simulink model "IEEE9Buses"  (R2024b)
settings: Solver=FixedStepAuto  StartTime=0  StopTime=5  FixedStep=1e-6  RelTol=1e-3
values from neighbouring files (symbols this model uses):
  SG_D_1_D = 0.01056    [SG9_parameters.m]
  SG_D_1_EnableSaturation = 0    [SG9_parameters.m]
  SG_D_1_f0 = 60    [SG9_parameters.m]
  SG_D_1_H = 7.5    [SG9_parameters.m]
  SG_D_1_K_A = 20    [SG9_parameters.m]
  SG_D_1_K_E = 1.000000e+1    (= 10)    [SG9_parameters.m]
  SG_D_1_K_F = 2.363    [SG9_parameters.m]
  SG_D_1_K_s = 5    [SG9_parameters.m]
  SG_D_1_R_a = 0.001088    [SG9_parameters.m]
  SG_D_1_S_A = 1    [SG9_parameters.m]
  SG_D_1_S_B = 0.103    [SG9_parameters.m]
  SG_D_1_S_N = 10.659857    [SG9_parameters.m]
  SG_D_1_SpeedPara = 200    [SG9_parameters.m]
  SG_D_1_T_0 = 0.720173    [SG9_parameters.m]
  SG_D_1_T_1 = 0.3    [SG9_parameters.m]
  SG_D_1_T_2 = 0.05    [SG9_parameters.m]
  SG_D_1_T_3 = 0.02    [SG9_parameters.m]
  SG_D_1_T_4 = 0.005    [SG9_parameters.m]
  SG_D_1_T_A = 0.02    [SG9_parameters.m]
  SG_D_1_T_dd = 8.000000e+0    (= 8)    [SG9_parameters.m]
  SG_D_1_T_ddd = 0.04    [SG9_parameters.m]
  SG_D_1_T_E = 0.314    [SG9_parameters.m]
  SG_D_1_T_F = 0.35    [SG9_parameters.m]
  SG_D_1_T_qd = 0.8    [SG9_parameters.m]
  SG_D_1_T_qdd = 0.02    [SG9_parameters.m]
  SG_D_1_T_speed = 0.1    [SG9_parameters.m]
  SG_D_1_T_w = 0.5    [SG9_parameters.m]
  SG_D_1_V_ref = 1.990276    [SG9_parameters.m]
  SG_D_1_w_ref = 376.991118    [SG9_parameters.m]
  SG_D_1_x_d = 1.9    [SG9_parameters.m]
  SG_D_1_x_dd = 0.302    [SG9_parameters.m]
  SG_D_1_x_ddd = 0.204    [SG9_parameters.m]
  SG_D_1_x_l = 0.05    [SG9_parameters.m]
  SG_D_1_x_q = 1.3    [SG9_parameters.m]
  SG_D_1_x_qd = 0.5    [SG9_parameters.m]
  SG_D_1_x_qdd = 0.3    [SG9_parameters.m]
  SG_D_2_D = 0.01056    [SG9_parameters.m]
  SG_D_2_EnableSaturation = 0    [SG9_parameters.m]
  SG_D_2_f0 = 60    [SG9_parameters.m]
  SG_D_2_H = 7.5    [SG9_parameters.m]
  SG_D_2_K_A = 20    [SG9_parameters.m]
  SG_D_2_K_E = 1.000000e+1    (= 10)    [SG9_parameters.m]
  SG_D_2_K_F = 2.363    [SG9_parameters.m]
  SG_D_2_K_s = 0.5    [SG9_parameters.m]
  SG_D_2_R_a = 0.001088    [SG9_parameters.m]
  SG_D_2_S_A = 1    [SG9_parameters.m]
  SG_D_2_S_B = 0.103    [SG9_parameters.m]
  SG_D_2_S_N = 10.659857    [SG9_parameters.m]
  SG_D_2_SpeedPara = 200    [SG9_parameters.m]
  SG_D_2_T_0 = 1.632913    [SG9_parameters.m]
  SG_D_2_T_1 = 0.2    [SG9_parameters.m]
  SG_D_2_T_2 = 0.05    [SG9_parameters.m]
  SG_D_2_T_3 = 0.02    [SG9_parameters.m]
  SG_D_2_T_4 = 0.005    [SG9_parameters.m]
  SG_D_2_T_A = 0.02    [SG9_parameters.m]
  SG_D_2_T_dd = 8.000000e+0    (= 8)    [SG9_parameters.m]
  SG_D_2_T_ddd = 0.04    [SG9_parameters.m]
  SG_D_2_T_E = 0.314    [SG9_parameters.m]
  SG_D_2_T_F = 0.35    [SG9_parameters.m]
  SG_D_2_T_qd = 0.8    [SG9_parameters.m]
  SG_D_2_T_qdd = 0.02    [SG9_parameters.m]
  SG_D_2_T_speed = 0.1    [SG9_parameters.m]
  SG_D_2_T_w = 0.5    [SG9_parameters.m]
  SG_D_2_V_ref = 2.662631    [SG9_parameters.m]
  SG_D_2_w_ref = 376.991118    [SG9_parameters.m]
  SG_D_2_x_d = 1.9    [SG9_parameters.m]
  SG_D_2_x_dd = 0.302    [SG9_parameters.m]
  SG_D_2_x_ddd = 0.204    [SG9_parameters.m]
  SG_D_2_x_l = 0.05    [SG9_parameters.m]
  SG_D_2_x_q = 1.3    [SG9_parameters.m]
  SG_D_2_x_qd = 0.5    [SG9_parameters.m]
  SG_D_2_x_qdd = 0.3    [SG9_parameters.m]
  SG_D_3_D = 0.01056    [SG9_parameters.m]
  SG_D_3_EnableSaturation = 0    [SG9_parameters.m]
  SG_D_3_f0 = 60    [SG9_parameters.m]
  SG_D_3_H = 7.5    [SG9_parameters.m]
  SG_D_3_K_A = 20    [SG9_parameters.m]
  SG_D_3_K_E = 1.000000e+1    (= 10)    [SG9_parameters.m]
  SG_D_3_K_F = 2.363    [SG9_parameters.m]
  SG_D_3_K_s = 0.5    [SG9_parameters.m]
  SG_D_3_R_a = 0.001088    [SG9_parameters.m]
  SG_D_3_S_A = 1    [SG9_parameters.m]
  SG_D_3_S_B = 0.103    [SG9_parameters.m]
  SG_D_3_S_N = 10.659857    [SG9_parameters.m]
  SG_D_3_SpeedPara = 200    [SG9_parameters.m]
  SG_D_3_T_0 = 0.850788    [SG9_parameters.m]
  SG_D_3_T_1 = 0.2    [SG9_parameters.m]
  SG_D_3_T_2 = 0.05    [SG9_parameters.m]
  SG_D_3_T_3 = 0.02    [SG9_parameters.m]
  SG_D_3_T_4 = 0.005    [SG9_parameters.m]
  SG_D_3_T_A = 0.02    [SG9_parameters.m]
  SG_D_3_T_dd = 8.000000e+0    (= 8)    [SG9_parameters.m]
  SG_D_3_T_ddd = 0.04    [SG9_parameters.m]
  SG_D_3_T_E = 0.314    [SG9_parameters.m]
  SG_D_3_T_F = 0.35    [SG9_parameters.m]
  SG_D_3_T_qd = 0.8    [SG9_parameters.m]
  SG_D_3_T_qdd = 0.02    [SG9_parameters.m]
  SG_D_3_T_speed = 0.1    [SG9_parameters.m]
  SG_D_3_T_w = 0.5    [SG9_parameters.m]
  SG_D_3_V_ref = 1.915682    [SG9_parameters.m]
  SG_D_3_w_ref = 376.991118    [SG9_parameters.m]
  SG_D_3_x_d = 1.9    [SG9_parameters.m]
  SG_D_3_x_dd = 0.302    [SG9_parameters.m]
  SG_D_3_x_ddd = 0.204    [SG9_parameters.m]
  SG_D_3_x_l = 0.05    [SG9_parameters.m]
  SG_D_3_x_q = 1.3    [SG9_parameters.m]
  SG_D_3_x_qd = 0.5    [SG9_parameters.m]
  SG_D_3_x_qdd = 0.3    [SG9_parameters.m]
(part 3 of 9)

== system IEEE9Buses/AC_1/d_vd_bus_2_block ==
  note: d_vd_bus_2 in SG9
      | $37699111.8430775\,\mathrm{id}_{\mathrm{bus},2}+376.991118430775\,\mathrm{vq}_{\mathrm{bus},2}$
      | Automatically generated on 2025-09-12 21:34:13 .
  Alge_id_bus_2_43cf4 : Inport
  State_vq_bus_2_cc1ad : Inport  Port=2
  Add_f2324 : Sum
  Constant_376.991118430775_c9407 : Constant  Value=376.991118430775
  Constant_37699111.8430775_545d6 : Constant  Value=37699111.8430775
  Product_1158d : Product
  Product_af620 : Product
  Blockout_d_vd_bus_2_ea113 : Outport
  wires:
  Constant_37699111.8430775_545d6/1 -> Product_af620/1
  Product_1158d/1 -> Add_f2324/2
  Alge_id_bus_2_43cf4/1 -> Product_af620/2
  Constant_376.991118430775_c9407/1 -> Product_1158d/1
  Product_af620/1 -> Add_f2324/1
  State_vq_bus_2_cc1ad/1 -> Product_1158d/2
  Add_f2324/1 -> Blockout_d_vd_bus_2_ea113/1

== system IEEE9Buses/AC_1/d_vd_bus_3_block ==
  note: d_vd_bus_3 in SG9
      | $37699111.8430775\,\mathrm{id}_{\mathrm{bus},3}+376.991118430775\,\mathrm{vq}_{\mathrm{bus},3}$
      | Automatically generated on 2025-09-12 21:34:14 .
  Alge_id_bus_3_37259 : Inport
  State_vq_bus_3_a84ef : Inport  Port=2
  Add_77a3c : Sum
  Constant_376.991118430775_0a76c : Constant  Value=376.991118430775
  Constant_37699111.8430775_f5c76 : Constant  Value=37699111.8430775
  Product_0f087 : Product
  Product_9c3ac : Product
  Blockout_d_vd_bus_3_60d94 : Outport
  wires:
  Constant_37699111.8430775_f5c76/1 -> Product_0f087/1
  Product_9c3ac/1 -> Add_77a3c/2
  Alge_id_bus_3_37259/1 -> Product_0f087/2
  Constant_376.991118430775_0a76c/1 -> Product_9c3ac/1
  Product_0f087/1 -> Add_77a3c/1
  State_vq_bus_3_a84ef/1 -> Product_9c3ac/2
  Add_77a3c/1 -> Blockout_d_vd_bus_3_60d94/1

== system IEEE9Buses/AC_1/d_vd_bus_4_block ==
  note: d_vd_bus_4 in SG9
      | $2257.43184689087\,\mathrm{id}_{\mathrm{bus},4}+376.991118430775\,\mathrm{vq}_{\mathrm{bus},4}$
      | Automatically generated on 2025-09-12 21:34:16 .
  Alge_id_bus_4_fcb80 : Inport
  State_vq_bus_4_57d81 : Inport  Port=2
  Add_d5196 : Sum
  Constant_2257.43184689087_07039 : Constant  Value=2257.43184689087
  Constant_376.991118430775_c2217 : Constant  Value=376.991118430775
  Product_11496 : Product
  Product_d7747 : Product
  Blockout_d_vd_bus_4_3a074 : Outport
  wires:
  Constant_2257.43184689087_07039/1 -> Product_11496/1
  Product_d7747/1 -> Add_d5196/2
  Alge_id_bus_4_fcb80/1 -> Product_11496/2
  Constant_376.991118430775_c2217/1 -> Product_d7747/1
  Product_11496/1 -> Add_d5196/1
  State_vq_bus_4_57d81/1 -> Product_d7747/2
  Add_d5196/1 -> Blockout_d_vd_bus_4_3a074/1

== system IEEE9Buses/AC_1/d_vd_bus_5_block ==
  note: d_vd_bus_5 in SG9
      | $1461.2058853906\,\mathrm{id}_{\mathrm{bus},5}+376.991118430775\,\mathrm{vq}_{\mathrm{bus},5}$
      | Automatically generated on 2025-09-12 21:34:17 .
  Alge_id_bus_5_7f9ce : Inport
  State_vq_bus_5_81ea0 : Inport  Port=2
  Add_dce3d : Sum
  Constant_1461.2058853906_6d3f5 : Constant  Value=1461.2058853906
  Constant_376.991118430775_eeefc : Constant  Value=376.991118430775
  Product_044f6 : Product
  Product_fe05c : Product
  Blockout_d_vd_bus_5_ffea6 : Outport
  wires:
  Constant_1461.2058853906_6d3f5/1 -> Product_fe05c/1
  Product_044f6/1 -> Add_dce3d/2
  Alge_id_bus_5_7f9ce/1 -> Product_fe05c/2
  Constant_376.991118430775_eeefc/1 -> Product_044f6/1
  Product_fe05c/1 -> Add_dce3d/1
  State_vq_bus_5_81ea0/1 -> Product_044f6/2
  Add_dce3d/1 -> Blockout_d_vd_bus_5_ffea6/1

== system IEEE9Buses/AC_1/d_vd_bus_6_block ==
  note: d_vd_bus_6 in SG9
      | $1329.77466818616\,\mathrm{id}_{\mathrm{bus},6}+376.991118430775\,\mathrm{vq}_{\mathrm{bus},6}$
      | Automatically generated on 2025-09-12 21:34:19 .
  Alge_id_bus_6_00f20 : Inport
  State_vq_bus_6_6b77a : Inport  Port=2
  Add_e78c5 : Sum
  Constant_1329.77466818616_73e1a : Constant  Value=1329.77466818616
  Constant_376.991118430775_ab125 : Constant  Value=376.991118430775
  Product_6150c : Product
  Product_b2199 : Product
  Blockout_d_vd_bus_6_a81cc : Outport
  wires:
  Constant_1329.77466818616_73e1a/1 -> Product_b2199/1
  Product_6150c/1 -> Add_e78c5/2
  Alge_id_bus_6_00f20/1 -> Product_b2199/2
  Constant_376.991118430775_ab125/1 -> Product_6150c/1
  Product_b2199/1 -> Add_e78c5/1
  State_vq_bus_6_6b77a/1 -> Product_6150c/2
  Add_e78c5/1 -> Blockout_d_vd_bus_6_a81cc/1

== system IEEE9Buses/AC_1/d_vd_bus_7_block ==
  note: d_vd_bus_7 in SG9
      | $2106.09563369148\,\mathrm{id}_{\mathrm{bus},7}+376.991118430775\,\mathrm{vq}_{\mathrm{bus},7}$
      | Automatically generated on 2025-09-12 21:34:20 .
  Alge_id_bus_7_c3139 : Inport
  State_vq_bus_7_fddcc : Inport  Port=2
  Add_c3fd4 : Sum
  Constant_2106.09563369148_db80e : Constant  Value=2106.09563369148
  Constant_376.991118430775_e3f6c : Constant  Value=376.991118430775
  Product_59e02 : Product
  Product_fc9d0 : Product
  Blockout_d_vd_bus_7_02e17 : Outport
  wires:
  Constant_2106.09563369148_db80e/1 -> Product_59e02/1
  Product_fc9d0/1 -> Add_c3fd4/2
  Alge_id_bus_7_c3139/1 -> Product_59e02/2
  Constant_376.991118430775_e3f6c/1 -> Product_fc9d0/1
  Product_59e02/1 -> Add_c3fd4/1
  State_vq_bus_7_fddcc/1 -> Product_fc9d0/2
  Add_c3fd4/1 -> Blockout_d_vd_bus_7_02e17/1

== system IEEE9Buses/AC_1/d_vd_bus_8_block ==
  note: d_vd_bus_8 in SG9
      | $1657.10381727813\,\mathrm{id}_{\mathrm{bus},8}+376.991118430775\,\mathrm{vq}_{\mathrm{bus},8}$
      | Automatically generated on 2025-09-12 21:34:22 .
  Alge_id_bus_8_fc0d0 : Inport
  State_vq_bus_8_879f9 : Inport  Port=2
  Add_b465b : Sum
  Constant_1657.10381727813_2791b : Constant  Value=1657.10381727813
  Constant_376.991118430775_c1762 : Constant  Value=376.991118430775
  Product_22d75 : Product
  Product_ba6e5 : Product
  Blockout_d_vd_bus_8_9b000 : Outport
  wires:
  Constant_1657.10381727813_2791b/1 -> Product_22d75/1
  Product_ba6e5/1 -> Add_b465b/2
  Alge_id_bus_8_fc0d0/1 -> Product_22d75/2
  Constant_376.991118430775_c1762/1 -> Product_ba6e5/1
  Product_22d75/1 -> Add_b465b/1
  State_vq_bus_8_879f9/1 -> Product_ba6e5/2
  Add_b465b/1 -> Blockout_d_vd_bus_8_9b000/1

== system IEEE9Buses/AC_1/d_vd_bus_9_block ==
  note: d_vd_bus_9 in SG9
      | $1564.27849971276\,\mathrm{id}_{\mathrm{bus},9}+376.991118430775\,\mathrm{vq}_{\mathrm{bus},9}$
      | Automatically generated on 2025-09-12 21:34:23 .
  Alge_id_bus_9_59e86 : Inport
  State_vq_bus_9_f7872 : Inport  Port=2
  Add_ffe46 : Sum
  Constant_1564.27849971276_b823b : Constant  Value=1564.27849971276
  Constant_376.991118430775_9e5bc : Constant  Value=376.991118430775
  Product_e292f : Product
  Product_fba56 : Product
  Blockout_d_vd_bus_9_33aa7 : Outport
  wires:
  Constant_1564.27849971276_b823b/1 -> Product_e292f/1
  Product_fba56/1 -> Add_ffe46/2
  Alge_id_bus_9_59e86/1 -> Product_e292f/2
  Constant_376.991118430775_9e5bc/1 -> Product_fba56/1
  Product_e292f/1 -> Add_ffe46/1
  State_vq_bus_9_f7872/1 -> Product_fba56/2
  Add_ffe46/1 -> Blockout_d_vd_bus_9_33aa7/1

== system IEEE9Buses/AC_1/d_vq_bus_1_block ==
  note: d_vq_bus_1 in SG9
      | $37699111.8430775\,\mathrm{iq}_{\mathrm{bus},1}-376.991118430775\,\mathrm{vd}_{\mathrm{bus},1}$
      | Automatically generated on 2025-09-12 21:34:12 .
  Alge_iq_bus_1_ef3c8 : Inport
  State_vd_bus_1_09d77 : Inport  Port=2
  Constant_376.991118430775_91f05 : Constant  Value=376.991118430775
  Constant_37699111.8430775_78d43 : Constant  Value=37699111.8430775
  Product_48b84 : Product
  Product_cddd7 : Product
  Subtract_09fbb : Sum  Inputs=+-
  Blockout_d_vq_bus_1_67500 : Outport
  wires:
  Constant_37699111.8430775_78d43/1 -> Product_cddd7/1
  Constant_376.991118430775_91f05/1 -> Product_48b84/1
  Alge_iq_bus_1_ef3c8/1 -> Product_cddd7/2
  State_vd_bus_1_09d77/1 -> Product_48b84/2
  Product_cddd7/1 -> Subtract_09fbb/1
  Product_48b84/1 -> Subtract_09fbb/2
  Subtract_09fbb/1 -> Blockout_d_vq_bus_1_67500/1

== system IEEE9Buses/AC_1/d_vq_bus_2_block ==
  note: d_vq_bus_2 in SG9
      | $37699111.8430775\,\mathrm{iq}_{\mathrm{bus},2}-376.991118430775\,\mathrm{vd}_{\mathrm{bus},2}$
      | Automatically generated on 2025-09-12 21:34:14 .
  Alge_iq_bus_2_d512d : Inport
  State_vd_bus_2_9829a : Inport  Port=2
  Constant_376.991118430775_711d0 : Constant  Value=376.991118430775
  Constant_37699111.8430775_cc7a6 : Constant  Value=37699111.8430775
  Product_2baa9 : Product
  Product_cb260 : Product
  Subtract_98bcc : Sum  Inputs=+-
  Blockout_d_vq_bus_2_b988a : Outport
  wires:
  Constant_37699111.8430775_cc7a6/1 -> Product_2baa9/1
  Constant_376.991118430775_711d0/1 -> Product_cb260/1
  Alge_iq_bus_2_d512d/1 -> Product_2baa9/2
  State_vd_bus_2_9829a/1 -> Product_cb260/2
  Product_2baa9/1 -> Subtract_98bcc/1
  Product_cb260/1 -> Subtract_98bcc/2
  Subtract_98bcc/1 -> Blockout_d_vq_bus_2_b988a/1

== system IEEE9Buses/AC_1/d_vq_bus_3_block ==
  note: d_vq_bus_3 in SG9
      | $37699111.8430775\,\mathrm{iq}_{\mathrm{bus},3}-376.991118430775\,\mathrm{vd}_{\mathrm{bus},3}$
      | Automatically generated on 2025-09-12 21:34:15 .
  Alge_iq_bus_3_4618e : Inport
  State_vd_bus_3_13373 : Inport  Port=2
  Constant_376.991118430775_82658 : Constant  Value=376.991118430775
  Constant_37699111.8430775_e2be2 : Constant  Value=37699111.8430775
  Product_0350b : Product
  Product_debd7 : Product
  Subtract_5e801 : Sum  Inputs=+-
  Blockout_d_vq_bus_3_efd63 : Outport
  wires:
  Constant_37699111.8430775_e2be2/1 -> Product_debd7/1
  Constant_376.991118430775_82658/1 -> Product_0350b/1
  Alge_iq_bus_3_4618e/1 -> Product_debd7/2
  State_vd_bus_3_13373/1 -> Product_0350b/2
  Product_debd7/1 -> Subtract_5e801/1
  Product_0350b/1 -> Subtract_5e801/2
  Subtract_5e801/1 -> Blockout_d_vq_bus_3_efd63/1

== system IEEE9Buses/AC_1/d_vq_bus_4_block ==
  note: d_vq_bus_4 in SG9
      | $2257.43184689087\,\mathrm{iq}_{\mathrm{bus},4}-376.991118430775\,\mathrm{vd}_{\mathrm{bus},4}$
      | Automatically generated on 2025-09-12 21:34:17 .
  Alge_iq_bus_4_4be37 : Inport
  State_vd_bus_4_edd2f : Inport  Port=2
  Constant_2257.43184689087_80e5c : Constant  Value=2257.43184689087
  Constant_376.991118430775_ec604 : Constant  Value=376.991118430775
  Product_aad31 : Product
  Product_bd912 : Product
  Subtract_6950c : Sum  Inputs=+-
  Blockout_d_vq_bus_4_2eed2 : Outport
  wires:
  Constant_2257.43184689087_80e5c/1 -> Product_bd912/1
  Constant_376.991118430775_ec604/1 -> Product_aad31/1
  Alge_iq_bus_4_4be37/1 -> Product_bd912/2
  State_vd_bus_4_edd2f/1 -> Product_aad31/2
  Product_bd912/1 -> Subtract_6950c/1
  Product_aad31/1 -> Subtract_6950c/2
  Subtract_6950c/1 -> Blockout_d_vq_bus_4_2eed2/1

== system IEEE9Buses/AC_1/d_vq_bus_5_block ==
  note: d_vq_bus_5 in SG9
      | $1461.2058853906\,\mathrm{iq}_{\mathrm{bus},5}-376.991118430775\,\mathrm{vd}_{\mathrm{bus},5}$
      | Automatically generated on 2025-09-12 21:34:18 .
  Alge_iq_bus_5_7cd16 : Inport
  State_vd_bus_5_232bf : Inport  Port=2
  Constant_1461.2058853906_f0ca2 : Constant  Value=1461.2058853906
  Constant_376.991118430775_0922f : Constant  Value=376.991118430775
  Product_2dcd7 : Product
  Product_91a48 : Product
  Subtract_696ec : Sum  Inputs=+-
  Blockout_d_vq_bus_5_a48d8 : Outport
  wires:
  Constant_1461.2058853906_f0ca2/1 -> Product_91a48/1
  Constant_376.991118430775_0922f/1 -> Product_2dcd7/1
  Alge_iq_bus_5_7cd16/1 -> Product_91a48/2
  State_vd_bus_5_232bf/1 -> Product_2dcd7/2
  Product_91a48/1 -> Subtract_696ec/1
  Product_2dcd7/1 -> Subtract_696ec/2
  Subtract_696ec/1 -> Blockout_d_vq_bus_5_a48d8/1

== system IEEE9Buses/AC_1/d_vq_bus_6_block ==
  note: d_vq_bus_6 in SG9
      | $1329.77466818616\,\mathrm{iq}_{\mathrm{bus},6}-376.991118430775\,\mathrm{vd}_{\mathrm{bus},6}$
      | Automatically generated on 2025-09-12 21:34:20 .
  Alge_iq_bus_6_c7a6f : Inport
  State_vd_bus_6_b0c85 : Inport  Port=2
  Constant_1329.77466818616_5019c : Constant  Value=1329.77466818616
  Constant_376.991118430775_e7c5b : Constant  Value=376.991118430775
  Product_08776 : Product
  Product_c21ee : Product
  Subtract_33230 : Sum  Inputs=+-
  Blockout_d_vq_bus_6_6730a : Outport
  wires:
  Constant_1329.77466818616_5019c/1 -> Product_08776/1
  Constant_376.991118430775_e7c5b/1 -> Product_c21ee/1
  Alge_iq_bus_6_c7a6f/1 -> Product_08776/2
  State_vd_bus_6_b0c85/1 -> Product_c21ee/2
  Product_08776/1 -> Subtract_33230/1
  Product_c21ee/1 -> Subtract_33230/2
  Subtract_33230/1 -> Blockout_d_vq_bus_6_6730a/1

== system IEEE9Buses/AC_1/d_vq_bus_7_block ==
  note: d_vq_bus_7 in SG9
      | $2106.09563369148\,\mathrm{iq}_{\mathrm{bus},7}-376.991118430775\,\mathrm{vd}_{\mathrm{bus},7}$
      | Automatically generated on 2025-09-12 21:34:21 .
  Alge_iq_bus_7_d2b8e : Inport
  State_vd_bus_7_25076 : Inport  Port=2
  Constant_2106.09563369148_c7572 : Constant  Value=2106.09563369148
  Constant_376.991118430775_ce9bf : Constant  Value=376.991118430775
  Product_412eb : Product
  Product_f2895 : Product
  Subtract_d5a52 : Sum  Inputs=+-
  Blockout_d_vq_bus_7_29dea : Outport
  wires:
  Constant_2106.09563369148_c7572/1 -> Product_412eb/1
  Product_f2895/1 -> Subtract_d5a52/2
  Alge_iq_bus_7_d2b8e/1 -> Product_412eb/2
  Constant_376.991118430775_ce9bf/1 -> Product_f2895/1
  Subtract_d5a52/1 -> Blockout_d_vq_bus_7_29dea/1
  State_vd_bus_7_25076/1 -> Product_f2895/2
  Product_412eb/1 -> Subtract_d5a52/1

== system IEEE9Buses/AC_1/d_vq_bus_8_block ==
  note: d_vq_bus_8 in SG9
      | $1657.10381727813\,\mathrm{iq}_{\mathrm{bus},8}-376.991118430775\,\mathrm{vd}_{\mathrm{bus},8}$
      | Automatically generated on 2025-09-12 21:34:23 .
  Alge_iq_bus_8_c37e6 : Inport
  State_vd_bus_8_17777 : Inport  Port=2
  Constant_1657.10381727813_86478 : Constant  Value=1657.10381727813
  Constant_376.991118430775_81401 : Constant  Value=376.991118430775
  Product_59b42 : Product
  Product_756dc : Product
  Subtract_6bda4 : Sum  Inputs=+-
  Blockout_d_vq_bus_8_0c63e : Outport
  wires:
  Constant_1657.10381727813_86478/1 -> Product_756dc/1
  Constant_376.991118430775_81401/1 -> Product_59b42/1
  Alge_iq_bus_8_c37e6/1 -> Product_756dc/2
  State_vd_bus_8_17777/1 -> Product_59b42/2
  Product_756dc/1 -> Subtract_6bda4/1
  Product_59b42/1 -> Subtract_6bda4/2
  Subtract_6bda4/1 -> Blockout_d_vq_bus_8_0c63e/1

== system IEEE9Buses/AC_1/d_vq_bus_9_block ==
  note: d_vq_bus_9 in SG9
      | $1564.27849971276\,\mathrm{iq}_{\mathrm{bus},9}-376.991118430775\,\mathrm{vd}_{\mathrm{bus},9}$
      | Automatically generated on 2025-09-12 21:34:24 .
  Alge_iq_bus_9_d9c5f : Inport
  State_vd_bus_9_b3036 : Inport  Port=2
  Constant_1564.27849971276_1fc79 : Constant  Value=1564.27849971276
  Constant_376.991118430775_6a9c1 : Constant  Value=376.991118430775
  Product_0f1cd : Product
  Product_eecd9 : Product
  Subtract_a27ba : Sum  Inputs=+-
  Blockout_d_vq_bus_9_7a2cb : Outport
  wires:
  Constant_1564.27849971276_1fc79/1 -> Product_0f1cd/1
  Constant_376.991118430775_6a9c1/1 -> Product_eecd9/1
  Alge_iq_bus_9_d9c5f/1 -> Product_0f1cd/2
  State_vd_bus_9_b3036/1 -> Product_eecd9/2
  Product_0f1cd/1 -> Subtract_a27ba/1
  Product_eecd9/1 -> Subtract_a27ba/2
  Subtract_a27ba/1 -> Blockout_d_vq_bus_9_7a2cb/1

== system IEEE9Buses/AC_1/id_bus_1_block ==
  note: id_bus_1 in SG9
      | $\mathrm{id}_{\mathrm{SG},D,1}-\mathrm{id}_{\mathrm{line},1,4}$
      | Automatically generated on 2025-09-12 21:34:50 .
  Input_id_SG_D_1_3262c : Inport
  State_id_line_1_4_5eb51 : Inport  Port=2
  Subtract_90a03 : Sum  Inputs=+-
  Blockout_id_bus_1_d304c : Outport
  wires:
  Input_id_SG_D_1_3262c/1 -> Subtract_90a03/1
  State_id_line_1_4_5eb51/1 -> Subtract_90a03/2
  Subtract_90a03/1 -> Blockout_id_bus_1_d304c/1

== system IEEE9Buses/AC_1/id_bus_2_block ==
  note: id_bus_2 in SG9
      | $\mathrm{id}_{\mathrm{SG},D,2}+\mathrm{id}_{\mathrm{line},8,2}$
      | Automatically generated on 2025-09-12 21:34:53 .
  Input_id_SG_D_2_e59e4 : Inport
  State_id_line_8_2_6326a : Inport  Port=2
  Add_90337 : Sum
  Blockout_id_bus_2_0c7b0 : Outport
  wires:
  Input_id_SG_D_2_e59e4/1 -> Add_90337/1
  State_id_line_8_2_6326a/1 -> Add_90337/2
  Add_90337/1 -> Blockout_id_bus_2_0c7b0/1

== system IEEE9Buses/AC_1/id_bus_3_block ==
  note: id_bus_3 in SG9
      | $\mathrm{id}_{\mathrm{SG},D,3}-\mathrm{id}_{\mathrm{line},3,6}$
      | Automatically generated on 2025-09-12 21:34:55 .
  Input_id_SG_D_3_5cb67 : Inport
  State_id_line_3_6_7876d : Inport  Port=2
  Subtract_b8691 : Sum  Inputs=+-
  Blockout_id_bus_3_8623b : Outport
  wires:
  Input_id_SG_D_3_5cb67/1 -> Subtract_b8691/1
  State_id_line_3_6_7876d/1 -> Subtract_b8691/2
  Subtract_b8691/1 -> Blockout_id_bus_3_8623b/1

== system IEEE9Buses/AC_1/id_bus_4_block ==
  note: id_bus_4 in SG9
      | $\mathrm{id}_{\mathrm{line},1,4}-\mathrm{id}_{\mathrm{line},4,5}+\mathrm{id}_{\mathrm{line},9,4}$
      | Automatically generated on 2025-09-12 21:34:57 .
  State_id_line_1_4_271d8 : Inport
  State_id_line_4_5_666cf : Inport  Port=2
  State_id_line_9_4_46c2c : Inport  Port=3
  Add_284bc : Sum
  Subtract_74750 : Sum  Inputs=+-
  Blockout_id_bus_4_7eb34 : Outport
  wires:
  State_id_line_9_4_46c2c/1 -> Add_284bc/2
  State_id_line_1_4_271d8/1 -> Subtract_74750/1
  State_id_line_4_5_666cf/1 -> Subtract_74750/2
  Subtract_74750/1 -> Add_284bc/1
  Add_284bc/1 -> Blockout_id_bus_4_7eb34/1

== system IEEE9Buses/AC_1/id_bus_5_block ==
  note: id_bus_5 in SG9
      | $\mathrm{id}_{\mathrm{line},4,5}-\mathrm{id}_{\mathrm{load},5}-\mathrm{id}_{\mathrm{line},5,6}$
      | Automatically generated on 2025-09-12 21:34:58 .
  State_id_load_5_1fb8c : Inport
  State_id_line_4_5_7fba6 : Inport  Port=2
  State_id_line_5_6_0d80f : Inport  Port=3
  Add_c924c : Sum
  Constant_-1_51db0 : Constant  Value=-1
  Product_7f1ab : Product
  Subtract_e8828 : Sum  Inputs=+-
  Blockout_id_bus_5_5017c : Outport
  wires:
  Subtract_e8828/1 -> Blockout_id_bus_5_5017c/1
  State_id_line_4_5_7fba6/1 -> Add_c924c/2
  Constant_-1_51db0/1 -> Product_7f1ab/1
  Add_c924c/1 -> Subtract_e8828/1
  State_id_load_5_1fb8c/1 -> Product_7f1ab/2
  Product_7f1ab/1 -> Add_c924c/1
  State_id_line_5_6_0d80f/1 -> Subtract_e8828/2

== system IEEE9Buses/AC_1/id_bus_6_block ==
  note: id_bus_6 in SG9
      | $\mathrm{id}_{\mathrm{line},3,6}+\mathrm{id}_{\mathrm{line},5,6}-\mathrm{id}_{\mathrm{line},6,7}$
      | Automatically generated on 2025-09-12 21:34:59 .
  State_id_line_3_6_8987c : Inport
  State_id_line_5_6_48a69 : Inport  Port=2
  State_id_line_6_7_545c3 : Inport  Port=3
  Add_21725 : Sum
  Subtract_edb02 : Sum  Inputs=+-
  Blockout_id_bus_6_b82c2 : Outport
  wires:
  State_id_line_6_7_545c3/1 -> Subtract_edb02/2
  State_id_line_3_6_8987c/1 -> Add_21725/1
  State_id_line_5_6_48a69/1 -> Add_21725/2
  Add_21725/1 -> Subtract_edb02/1
  Subtract_edb02/1 -> Blockout_id_bus_6_b82c2/1

== system IEEE9Buses/AC_1/id_bus_7_block ==
  note: id_bus_7 in SG9
      | $\mathrm{id}_{\mathrm{line},6,7}-\mathrm{id}_{\mathrm{load},7}-\mathrm{id}_{\mathrm{line},7,8}$
      | Automatically generated on 2025-09-12 21:35:01 .
  State_id_load_7_766eb : Inport
  State_id_line_6_7_e269f : Inport  Port=2
  State_id_line_7_8_76347 : Inport  Port=3
  Add_5aa98 : Sum
  Constant_-1_3d25f : Constant  Value=-1
  Product_22e44 : Product
  Subtract_98307 : Sum  Inputs=+-
  Blockout_id_bus_7_881bd : Outport
  wires:
  Subtract_98307/1 -> Blockout_id_bus_7_881bd/1
  State_id_line_6_7_e269f/1 -> Add_5aa98/2
  Constant_-1_3d25f/1 -> Product_22e44/1
  Add_5aa98/1 -> Subtract_98307/1
  State_id_load_7_766eb/1 -> Product_22e44/2
  Product_22e44/1 -> Add_5aa98/1
  State_id_line_7_8_76347/1 -> Subtract_98307/2

== system IEEE9Buses/AC_1/id_bus_8_block ==
  note: id_bus_8 in SG9
      | $\mathrm{id}_{\mathrm{line},7,8}-\mathrm{id}_{\mathrm{line},8,2}-\mathrm{id}_{\mathrm{line},8,9}$
      | Automatically generated on 2025-09-12 21:35:02 .
  State_id_line_7_8_ffd1a : Inport
  State_id_line_8_2_3b688 : Inport  Port=2
  State_id_line_8_9_87c38 : Inport  Port=3
  Subtract_91b76 : Sum  Inputs=+-
  Subtract_aa8d0 : Sum  Inputs=+-
  Blockout_id_bus_8_27f10 : Outport
  wires:
  State_id_line_8_9_87c38/1 -> Subtract_91b76/2
  State_id_line_7_8_ffd1a/1 -> Subtract_aa8d0/1
  State_id_line_8_2_3b688/1 -> Subtract_aa8d0/2
  Subtract_aa8d0/1 -> Subtract_91b76/1
  Subtract_91b76/1 -> Blockout_id_bus_8_27f10/1

== system IEEE9Buses/AC_1/id_bus_9_block ==
  note: id_bus_9 in SG9
      | $\mathrm{id}_{\mathrm{line},8,9}-\mathrm{id}_{\mathrm{load},9}-\mathrm{id}_{\mathrm{line},9,4}$
      | Automatically generated on 2025-09-12 21:35:03 .
  State_id_load_9_21730 : Inport
  State_id_line_8_9_2ef8e : Inport  Port=2
  State_id_line_9_4_80368 : Inport  Port=3
  Add_7e365 : Sum
  Constant_-1_9b3fa : Constant  Value=-1
  Product_e1c40 : Product
  Subtract_404db : Sum  Inputs=+-
  Blockout_id_bus_9_52737 : Outport
  wires:
  Subtract_404db/1 -> Blockout_id_bus_9_52737/1
  State_id_line_8_9_2ef8e/1 -> Add_7e365/2
  Constant_-1_9b3fa/1 -> Product_e1c40/1
  Add_7e365/1 -> Subtract_404db/1
  State_id_load_9_21730/1 -> Product_e1c40/2
  Product_e1c40/1 -> Add_7e365/1
  State_id_line_9_4_80368/1 -> Subtract_404db/2

== system IEEE9Buses/AC_1/iq_bus_1_block ==
  note: iq_bus_1 in SG9
      | $\mathrm{iq}_{\mathrm{SG},D,1}-\mathrm{iq}_{\mathrm{line},1,4}$
      | Automatically generated on 2025-09-12 21:34:51 .
  Input_iq_SG_D_1_ca28f : Inport
  State_iq_line_1_4_8883d : Inport  Port=2
  Subtract_daff4 : Sum  Inputs=+-
  Blockout_iq_bus_1_b29d9 : Outport
  wires:
  Input_iq_SG_D_1_ca28f/1 -> Subtract_daff4/1
  State_iq_line_1_4_8883d/1 -> Subtract_daff4/2
  Subtract_daff4/1 -> Blockout_iq_bus_1_b29d9/1

== system IEEE9Buses/AC_1/iq_bus_2_block ==
  note: iq_bus_2 in SG9
      | $\mathrm{iq}_{\mathrm{SG},D,2}+\mathrm{iq}_{\mathrm{line},8,2}$
      | Automatically generated on 2025-09-12 21:34:53 .
  Input_iq_SG_D_2_644f3 : Inport
  State_iq_line_8_2_4a7a6 : Inport  Port=2
  Add_813f5 : Sum
  Blockout_iq_bus_2_e5997 : Outport
  wires:
  Input_iq_SG_D_2_644f3/1 -> Add_813f5/1
  State_iq_line_8_2_4a7a6/1 -> Add_813f5/2
  Add_813f5/1 -> Blockout_iq_bus_2_e5997/1

== system IEEE9Buses/AC_1/iq_bus_3_block ==
  note: iq_bus_3 in SG9
      | $\mathrm{iq}_{\mathrm{SG},D,3}-\mathrm{iq}_{\mathrm{line},3,6}$
      | Automatically generated on 2025-09-12 21:34:56 .
  Input_iq_SG_D_3_d199a : Inport
  State_iq_line_3_6_8aa40 : Inport  Port=2
  Subtract_d75df : Sum  Inputs=+-
  Blockout_iq_bus_3_7a5f4 : Outport
  wires:
  Input_iq_SG_D_3_d199a/1 -> Subtract_d75df/1
  State_iq_line_3_6_8aa40/1 -> Subtract_d75df/2
  Subtract_d75df/1 -> Blockout_iq_bus_3_7a5f4/1

== system IEEE9Buses/AC_1/iq_bus_4_block ==
  note: iq_bus_4 in SG9
      | $\mathrm{iq}_{\mathrm{line},1,4}-\mathrm{iq}_{\mathrm{line},4,5}+\mathrm{iq}_{\mathrm{line},9,4}$
      | Automatically generated on 2025-09-12 21:34:57 .
  State_iq_line_1_4_f419e : Inport
  State_iq_line_4_5_eba88 : Inport  Port=2
  State_iq_line_9_4_7b513 : Inport  Port=3
  Add_3ef12 : Sum
  Subtract_a9e9f : Sum  Inputs=+-
  Blockout_iq_bus_4_66e6a : Outport
  wires:
  State_iq_line_1_4_f419e/1 -> Subtract_a9e9f/1
  State_iq_line_4_5_eba88/1 -> Subtract_a9e9f/2
  Subtract_a9e9f/1 -> Add_3ef12/1
  State_iq_line_9_4_7b513/1 -> Add_3ef12/2
  Add_3ef12/1 -> Blockout_iq_bus_4_66e6a/1

== system IEEE9Buses/AC_1/iq_bus_5_block ==
  note: iq_bus_5 in SG9
      | $\mathrm{iq}_{\mathrm{line},4,5}-\mathrm{iq}_{\mathrm{load},5}-\mathrm{iq}_{\mathrm{line},5,6}$
      | Automatically generated on 2025-09-12 21:34:59 .
  State_iq_load_5_4f98c : Inport
  State_iq_line_4_5_8b006 : Inport  Port=2
  State_iq_line_5_6_de832 : Inport  Port=3
  Add_02e77 : Sum
  Constant_-1_71d1b : Constant  Value=-1
  Product_b953c : Product
  Subtract_08be3 : Sum  Inputs=+-
  Blockout_iq_bus_5_cd3aa : Outport
  wires:
  Subtract_08be3/1 -> Blockout_iq_bus_5_cd3aa/1
  State_iq_line_4_5_8b006/1 -> Add_02e77/2
  Constant_-1_71d1b/1 -> Product_b953c/1
  State_iq_load_5_4f98c/1 -> Product_b953c/2
  Product_b953c/1 -> Add_02e77/1
  Add_02e77/1 -> Subtract_08be3/1
  State_iq_line_5_6_de832/1 -> Subtract_08be3/2

== system IEEE9Buses/AC_1/iq_bus_6_block ==
  note: iq_bus_6 in SG9
      | $\mathrm{iq}_{\mathrm{line},3,6}+\mathrm{iq}_{\mathrm{line},5,6}-\mathrm{iq}_{\mathrm{line},6,7}$
      | Automatically generated on 2025-09-12 21:35:00 .
  State_iq_line_3_6_58a90 : Inport
  State_iq_line_5_6_012cd : Inport  Port=2
  State_iq_line_6_7_0570d : Inport  Port=3
  Add_3b3d7 : Sum
  Subtract_2de7b : Sum  Inputs=+-
  Blockout_iq_bus_6_e51e3 : Outport
  wires:
  State_iq_line_3_6_58a90/1 -> Add_3b3d7/1
  State_iq_line_5_6_012cd/1 -> Add_3b3d7/2
  Add_3b3d7/1 -> Subtract_2de7b/1
  State_iq_line_6_7_0570d/1 -> Subtract_2de7b/2
  Subtract_2de7b/1 -> Blockout_iq_bus_6_e51e3/1

== system IEEE9Buses/AC_1/iq_bus_7_block ==
  note: iq_bus_7 in SG9
      | $\mathrm{iq}_{\mathrm{line},6,7}-\mathrm{iq}_{\mathrm{load},7}-\mathrm{iq}_{\mathrm{line},7,8}$
      | Automatically generated on 2025-09-12 21:35:01 .
  State_iq_load_7_0f831 : Inport
  State_iq_line_6_7_a92f3 : Inport  Port=2
  State_iq_line_7_8_2c1c0 : Inport  Port=3
  Add_b0ba0 : Sum
  Constant_-1_dd50e : Constant  Value=-1
  Product_e06f3 : Product
  Subtract_ab063 : Sum  Inputs=+-
  Blockout_iq_bus_7_33867 : Outport
  wires:
  Subtract_ab063/1 -> Blockout_iq_bus_7_33867/1
  State_iq_line_6_7_a92f3/1 -> Add_b0ba0/2
  Constant_-1_dd50e/1 -> Product_e06f3/1
  State_iq_load_7_0f831/1 -> Product_e06f3/2
  Product_e06f3/1 -> Add_b0ba0/1
  Add_b0ba0/1 -> Subtract_ab063/1
  State_iq_line_7_8_2c1c0/1 -> Subtract_ab063/2

== system IEEE9Buses/AC_1/iq_bus_8_block ==
  note: iq_bus_8 in SG9
      | $\mathrm{iq}_{\mathrm{line},7,8}-\mathrm{iq}_{\mathrm{line},8,2}-\mathrm{iq}_{\mathrm{line},8,9}$
      | Automatically generated on 2025-09-12 21:35:02 .
  State_iq_line_7_8_aee75 : Inport
  State_iq_line_8_2_9e1b5 : Inport  Port=2
  State_iq_line_8_9_ce938 : Inport  Port=3
  Subtract_38bfc : Sum  Inputs=+-
  Subtract_4a1f1 : Sum  Inputs=+-
  Blockout_iq_bus_8_e3563 : Outport
  wires:
  State_iq_line_7_8_aee75/1 -> Subtract_38bfc/1
  State_iq_line_8_2_9e1b5/1 -> Subtract_38bfc/2
  Subtract_38bfc/1 -> Subtract_4a1f1/1
  State_iq_line_8_9_ce938/1 -> Subtract_4a1f1/2
  Subtract_4a1f1/1 -> Blockout_iq_bus_8_e3563/1

== system IEEE9Buses/AC_1/iq_bus_9_block ==
  note: iq_bus_9 in SG9
      | $\mathrm{iq}_{\mathrm{line},8,9}-\mathrm{iq}_{\mathrm{load},9}-\mathrm{iq}_{\mathrm{line},9,4}$
      | Automatically generated on 2025-09-12 21:35:04 .
  State_iq_load_9_c7d1b : Inport
  State_iq_line_8_9_c4804 : Inport  Port=2
  State_iq_line_9_4_0e87b : Inport  Port=3
  Add_08581 : Sum
  Constant_-1_c81b7 : Constant  Value=-1
  Product_af021 : Product
  Subtract_950eb : Sum  Inputs=+-
  Blockout_iq_bus_9_40080 : Outport
  wires:
  Subtract_950eb/1 -> Blockout_iq_bus_9_40080/1
  State_iq_line_8_9_c4804/1 -> Add_08581/2
  Constant_-1_c81b7/1 -> Product_af021/1
  State_iq_load_9_c7d1b/1 -> Product_af021/2
  Product_af021/1 -> Add_08581/1
  Add_08581/1 -> Subtract_950eb/1
  State_iq_line_9_4_0e87b/1 -> Subtract_950eb/2

== system IEEE9Buses/AC_1/vd_bus_1_out_block ==
  note: vd_bus_1_out in SG9
      | $\mathrm{vd}_{\mathrm{bus},1}$
      | Automatically generated on 2025-09-12 21:34:49 .
  State_vd_bus_1_30b4d : Inport
  Blockout_vd_bus_1_out_0277b : Outport
  wires:
  State_vd_bus_1_30b4d/1 -> Blockout_vd_bus_1_out_0277b/1

== system IEEE9Buses/AC_1/vd_bus_2_out_block ==
  note: vd_bus_2_out in SG9
      | $\mathrm{vd}_{\mathrm{bus},2}$
      | Automatically generated on 2025-09-12 21:34:52 .
  State_vd_bus_2_7ad9e : Inport
  Blockout_vd_bus_2_out_05523 : Outport
  wires:
  State_vd_bus_2_7ad9e/1 -> Blockout_vd_bus_2_out_05523/1

== system IEEE9Buses/AC_1/vd_bus_3_out_block ==
  note: vd_bus_3_out in SG9
      | $\mathrm{vd}_{\mathrm{bus},3}$
      | Automatically generated on 2025-09-12 21:34:54 .
  State_vd_bus_3_69656 : Inport
  Blockout_vd_bus_3_out_02f53 : Outport
  wires:
  State_vd_bus_3_69656/1 -> Blockout_vd_bus_3_out_02f53/1

== system IEEE9Buses/AC_1/vq_bus_1_out_block ==
  note: vq_bus_1_out in SG9
      | $\mathrm{vq}_{\mathrm{bus},1}$
      | Automatically generated on 2025-09-12 21:34:49 .
  State_vq_bus_1_02b5e : Inport
  Blockout_vq_bus_1_out_8292c : Outport
  wires:
  State_vq_bus_1_02b5e/1 -> Blockout_vq_bus_1_out_8292c/1

== system IEEE9Buses/AC_1/vq_bus_2_out_block ==
  note: vq_bus_2_out in SG9
      | $\mathrm{vq}_{\mathrm{bus},2}$
      | Automatically generated on 2025-09-12 21:34:52 .
  State_vq_bus_2_14eae : Inport
  Blockout_vq_bus_2_out_74947 : Outport
  wires:
  State_vq_bus_2_14eae/1 -> Blockout_vq_bus_2_out_74947/1

== system IEEE9Buses/AC_1/vq_bus_3_out_block ==
  note: vq_bus_3_out in SG9
      | $\mathrm{vq}_{\mathrm{bus},3}$
      | Automatically generated on 2025-09-12 21:34:55 .
  State_vq_bus_3_9203b : Inport
  Blockout_vq_bus_3_out_11dc3 : Outport
  wires:
  State_vq_bus_3_9203b/1 -> Blockout_vq_bus_3_out_11dc3/1

== system IEEE9Buses/SG_D_1/T_e_SG_D_1_block ==
  note: T_e_SG_D_1 in SG9
      | $-\frac{\psi _{d,\mathrm{SG},D,1}\,\left(\psi _{q,\mathrm{SG},D,1}+\frac{\psi _{\mathrm{gq},\mathrm{SG},D,1}\,\left(x_{l}-x_{\mathrm{qdd}}\right)}{x_{l}-x_{\mathrm{qd}}}+\frac{\psi _{\mathrm{kq},\mathrm{SG},D,1}\,\left(x_{\mathrm{qd}}-x_{\mathrm{qdd}}\right)}{x_{l}-x_{\mathrm{qd}}}\right)}{x_{\mathrm{qdd}}}-\frac{\psi _{q,\mathrm{SG},D,1}\,\left(\frac{\psi _{\mathrm{1d},\mathrm{SG},D,1}\,\left(x_{\mathrm{dd}}-x_{\mathrm{ddd}}\right)}{x_{\mathrm{dd}}-x_{l}}-\psi _{d,\mathrm{SG},D,1}+\frac{\psi _{\mathrm{fd},\mathrm{SG},D,1}\,\left(x_{\mathrm{ddd}}-x_{l}\right)}{x_{\mathrm{dd}}-x_{l}}\right)}{x_{\mathrm{ddd}}}$
      | Automatically generated on 2025-09-12 21:31:47 .
  State_psi_d_SG_D_1_0962a : Inport
  State_psi_gq_SG_D_1_b4b18 : Inport  Port=2
  State_psi_kq_SG_D_1_b55ca : Inport  Port=3
  State_psi_q_SG_D_1_5bbe1 : Inport  Port=4
  State_psi_q_SG_D_1_be59e : Inport  Port=5
  State_psi_1d_SG_D_1_94903 : Inport  Port=6
  State_psi_d_SG_D_1_5996b : Inport  Port=7
  State_psi_fd_SG_D_1_1100d : Inport  Port=8
  Add_1b04a : Sum
  Add_49a3f : Sum
  Add_8fcaf : Sum
  Add_bb93d : Sum
  Add_c5540 : Sum
  Add_cd011 : Sum
  Constant_-1_0fac1 : Constant  Value=-1
  Constant_-1_11887 : Constant  Value=-1
  Constant_-1_5095d : Constant  Value=-1
  Constant_-1_67393 : Constant  Value=-1
  Constant_-1_ff001 : Constant  Value=-1
  Constant_x_dd_0a5f9 : Constant  Value=x_dd
  Constant_x_dd_1a143 : Constant  Value=x_dd
  Constant_x_dd_d3647 : Constant  Value=x_dd
  Constant_x_ddd_0a7df : Constant  Value=x_ddd
  Constant_x_ddd_3d1ac : Constant  Value=x_ddd
  Constant_x_ddd_bee41 : Constant  Value=x_ddd
  Constant_x_l_0af48 : Constant  Value=x_l
  Constant_x_l_36fe6 : Constant  Value=x_l
  Constant_x_l_3a877 : Constant  Value=x_l
  Constant_x_l_591cf : Constant  Value=x_l
  Constant_x_l_a665b : Constant  Value=x_l
  Constant_x_l_f5a51 : Constant  Value=x_l
  Constant_x_qd_13d21 : Constant  Value=x_qd
  Constant_x_qd_160ff : Constant  Value=x_qd
  Constant_x_qd_61dee : Constant  Value=x_qd
  Constant_x_qdd_14e72 : Constant  Value=x_qdd
  Constant_x_qdd_7a81b : Constant  Value=x_qdd
  Constant_x_qdd_949d0 : Constant  Value=x_qdd
  Divide_0f8fa : Product  Inputs=*/
  Divide_2d360 : Product  Inputs=*/
  Divide_38438 : Product  Inputs=*/
  Divide_b5984 : Product  Inputs=*/
  Divide_eae6b : Product  Inputs=*/
  Divide_ec87e : Product  Inputs=*/
  Product_0bf95 : Product
  Product_333b9 : Product
  Product_527a6 : Product
  Product_87aa7 : Product
  Product_8b9b7 : Product
  Product_aff61 : Product
  Product_b860c : Product
  Product_b8eef : Product
  Product_bdae3 : Product
  Product_c1012 : Product
  Product_fe8c6 : Product
  Subtract_0db52 : Sum  Inputs=+-
  Subtract_7421d : Sum  Inputs=+-
  Subtract_86223 : Sum  Inputs=+-
  Subtract_9d169 : Sum  Inputs=+-
  Subtract_9e53a : Sum  Inputs=+-
  Subtract_dd774 : Sum  Inputs=+-
  Subtract_eb507 : Sum  Inputs=+-
  Blockout_T_e_SG_D_1_6e908 : Outport
  wires:
  Product_aff61/1 -> Divide_ec87e/1
  Product_c1012/1 -> Add_8fcaf/1
  Divide_ec87e/1 -> Subtract_7421d/1
  Constant_-1_0fac1/1 -> Product_c1012/1
  Constant_x_l_a665b/1 -> Product_c1012/2
  Constant_x_qdd_949d0/1 -> Add_8fcaf/2
  Constant_x_qd_61dee/1 -> Subtract_86223/1
  Constant_-1_11887/1 -> Product_b860c/1
  Constant_x_qdd_14e72/1 -> Divide_0f8fa/2
  Constant_x_qdd_7a81b/1 -> Subtract_86223/2
  State_psi_q_SG_D_1_be59e/1 -> Product_bdae3/1
  Constant_x_dd_1a143/1 -> Subtract_9d169/1
  Constant_x_l_0af48/1 -> Product_b860c/2
  Subtract_9d169/1 -> Product_87aa7/2
  Constant_-1_5095d/1 -> Product_fe8c6/1
  Constant_x_l_36fe6/1 -> Product_fe8c6/2
  Subtract_0db52/1 -> Product_bdae3/2
  State_psi_q_SG_D_1_5bbe1/1 -> Add_c5540/2
  Constant_-1_ff001/1 -> Product_0bf95/1
  State_psi_1d_SG_D_1_94903/1 -> Product_0bf95/2
  Constant_x_ddd_3d1ac/1 -> Subtract_9d169/2
  State_psi_gq_SG_D_1_b4b18/1 -> Product_aff61/1
  Add_8fcaf/1 -> Product_aff61/2
  Product_b860c/1 -> Add_1b04a/1
  Product_333b9/1 -> Product_b8eef/1
  Constant_x_qd_13d21/1 -> Add_1b04a/2
  Product_87aa7/1 -> Divide_eae6b/1
  State_psi_kq_SG_D_1_b55ca/1 -> Product_8b9b7/1
  Add_1b04a/1 -> Divide_ec87e/2
  Subtract_86223/1 -> Product_8b9b7/2
  Product_fe8c6/1 -> Add_49a3f/1
  Constant_x_qd_160ff/1 -> Add_49a3f/2
  Product_8b9b7/1 -> Divide_38438/1
  Product_0bf95/1 -> Product_87aa7/1
  Constant_x_dd_d3647/1 -> Subtract_9e53a/1
  Constant_x_l_3a877/1 -> Subtract_9e53a/2
  Constant_x_ddd_bee41/1 -> Subtract_dd774/1
  Product_bdae3/1 -> Divide_2d360/1
  Constant_x_l_591cf/1 -> Subtract_dd774/2
  Divide_0f8fa/1 -> Add_bb93d/1
  Product_b8eef/1 -> Divide_0f8fa/1
  Add_49a3f/1 -> Divide_38438/2
  Subtract_7421d/1 -> Add_c5540/1
  Divide_38438/1 -> Subtract_7421d/2
  Subtract_9e53a/1 -> Divide_eae6b/2
  State_psi_fd_SG_D_1_1100d/1 -> Product_527a6/1
  Constant_x_ddd_0a7df/1 -> Divide_2d360/2
  Subtract_dd774/1 -> Product_527a6/2
  Constant_x_dd_0a5f9/1 -> Subtract_eb507/1
  Constant_x_l_f5a51/1 -> Subtract_eb507/2
  Divide_eae6b/1 -> Add_cd011/1
  Add_cd011/1 -> Subtract_0db52/1
  State_psi_d_SG_D_1_5996b/1 -> Add_cd011/2
  Product_527a6/1 -> Divide_b5984/1
  Subtract_eb507/1 -> Divide_b5984/2
  Constant_-1_67393/1 -> Product_333b9/1
  State_psi_d_SG_D_1_0962a/1 -> Product_333b9/2
  Divide_b5984/1 -> Subtract_0db52/2
  Add_c5540/1 -> Product_b8eef/2
  Divide_2d360/1 -> Add_bb93d/2
  Add_bb93d/1 -> Blockout_T_e_SG_D_1_6e908/1

== system IEEE9Buses/SG_D_1/d_E_fd_SG_D_1_block ==
  note: d_E_fd_SG_D_1 in SG9
      | $\frac{V_{f,\mathrm{SG},D,1}-E_{\mathrm{fd},\mathrm{SG},D,1}\,K_{E}}{T_{E}}$
      | Automatically generated on 2025-09-12 21:31:30 .
  State_E_fd_SG_D_1_82d72 : Inport
  State_V_f_SG_D_1_23896 : Inport  Port=2
  Add_cc2aa : Sum
  Constant_-1_60bb5 : Constant  Value=-1
  Constant_K_E_bab65 : Constant  Value=K_E
  Constant_T_E_ec6db : Constant  Value=T_E
  Divide_ae0d3 : Product  Inputs=*/
  Product_4f692 : Product
  Product_c6492 : Product
  Blockout_d_E_fd_SG_D_1_51f8a : Outport
  wires:
  Add_cc2aa/1 -> Divide_ae0d3/1
  Constant_-1_60bb5/1 -> Product_4f692/1
  State_E_fd_SG_D_1_82d72/1 -> Product_4f692/2
  Product_4f692/1 -> Product_c6492/1
  Constant_K_E_bab65/1 -> Product_c6492/2
  Product_c6492/1 -> Add_cc2aa/1
  Constant_T_E_ec6db/1 -> Divide_ae0d3/2
  State_V_f_SG_D_1_23896/1 -> Add_cc2aa/2
  Divide_ae0d3/1 -> Blockout_d_E_fd_SG_D_1_51f8a/1

== system IEEE9Buses/SG_D_1/d_Px_1_SG_D_1_block ==
  note: d_Px_1_SG_D_1 in SG9
      | $\frac{w_{\mathrm{SG},D,1}-2\,\pi \,f_{0}}{T_{w}}-\frac{\mathrm{Px}_{1,\mathrm{SG},D,1}}{T_{w}}$
      | Automatically generated on 2025-09-12 21:31:31 .
  State_Px_1_SG_D_1_0d11e : Inport
  State_w_SG_D_1_abb95 : Inport  Port=2
  Add_5b772 : Sum
  Add_c551c : Sum
  Constant_-1_499ec : Constant  Value=-1
  Constant_-2.0_3f3c7 : Constant  Value=-2.0
  Constant_T_w_81e01 : Constant  Value=T_w
  Constant_T_w_dd83f : Constant  Value=T_w
  Constant_f0_71ba1 : Constant  Value=f0
  Constant_pi_42c04 : Constant  Value=pi
  Divide_2fdde : Product  Inputs=*/
  Divide_914c0 : Product  Inputs=*/
  Product_bb841 : Product
  Product_c3fb5 : Product
  Product_ebf0a : Product
  Blockout_d_Px_1_SG_D_1_cf474 : Outport
  wires:
  Add_c551c/1 -> Blockout_d_Px_1_SG_D_1_cf474/1
  Constant_-2.0_3f3c7/1 -> Product_c3fb5/1
  Product_bb841/1 -> Divide_914c0/1
  State_w_SG_D_1_abb95/1 -> Add_5b772/2
  Constant_-1_499ec/1 -> Product_bb841/1
  Constant_f0_71ba1/1 -> Product_ebf0a/2
  Constant_pi_42c04/1 -> Product_c3fb5/2
  Product_ebf0a/1 -> Add_5b772/1
  Product_c3fb5/1 -> Product_ebf0a/1
  State_Px_1_SG_D_1_0d11e/1 -> Product_bb841/2
  Constant_T_w_81e01/1 -> Divide_914c0/2
  Add_5b772/1 -> Divide_2fdde/1
  Constant_T_w_dd83f/1 -> Divide_2fdde/2
  Divide_914c0/1 -> Add_c551c/1
  Divide_2fdde/1 -> Add_c551c/2

== system IEEE9Buses/SG_D_1/d_Px_2_SG_D_1_block ==
  note: d_Px_2_SG_D_1 in SG9
      | $\frac{\mathrm{Px}_{1,\mathrm{SG},D,1}-T_{2}\,\left(\frac{\mathrm{Px}_{1,\mathrm{SG},D,1}}{T_{w}}-\frac{w_{\mathrm{SG},D,1}-2\,\pi \,f_{0}}{T_{w}}\right)}{T_{1}}-\frac{\mathrm{Px}_{2,\mathrm{SG},D,1}}{T_{1}}$
      | Automatically generated on 2025-09-12 21:31:33 .
  State_Px_2_SG_D_1_42d3f : Inport
  State_Px_1_SG_D_1_862b1 : Inport  Port=2
  State_Px_1_SG_D_1_1d3a0 : Inport  Port=3
  State_w_SG_D_1_fc7e0 : Inport  Port=4
  Add_26b4f : Sum
  Add_6853f : Sum
  Add_adb86 : Sum
  Add_d978a : Sum
  Constant_-1_74494 : Constant  Value=-1
  Constant_-1_7f639 : Constant  Value=-1
  Constant_-2.0_1314f : Constant  Value=-2.0
  Constant_T_1_7fbbd : Constant  Value=T_1
  Constant_T_1_c3252 : Constant  Value=T_1
  Constant_T_2_98f2f : Constant  Value=T_2
  Constant_T_w_57f06 : Constant  Value=T_w
  Constant_T_w_a5177 : Constant  Value=T_w
  Constant_f0_46377 : Constant  Value=f0
  Constant_pi_d0684 : Constant  Value=pi
  Divide_4af5b : Product  Inputs=*/
  Divide_6a425 : Product  Inputs=*/
  Divide_a35e7 : Product  Inputs=*/
  Divide_d781c : Product  Inputs=*/
  Product_2faf8 : Product
  Product_3aa50 : Product
  Product_81a86 : Product
  Product_8b2f7 : Product
  Product_e53b9 : Product
  Blockout_d_Px_2_SG_D_1_42534 : Outport
  wires:
  Constant_-2.0_1314f/1 -> Product_8b2f7/1
  State_w_SG_D_1_fc7e0/1 -> Add_adb86/2
  Constant_f0_46377/1 -> Product_81a86/2
  Constant_pi_d0684/1 -> Product_8b2f7/2
  Add_26b4f/1 -> Product_e53b9/2
  Product_81a86/1 -> Add_adb86/1
  Divide_a35e7/1 -> Add_26b4f/1
  Product_8b2f7/1 -> Product_81a86/1
  Constant_T_w_a5177/1 -> Divide_a35e7/2
  Constant_-1_7f639/1 -> Product_3aa50/1
  State_Px_1_SG_D_1_1d3a0/1 -> Product_3aa50/2
  Divide_6a425/1 -> Add_d978a/1
  Product_3aa50/1 -> Divide_a35e7/1
  Add_adb86/1 -> Divide_4af5b/1
  Constant_T_w_57f06/1 -> Divide_4af5b/2
  Divide_4af5b/1 -> Add_26b4f/2
  Constant_T_2_98f2f/1 -> Product_e53b9/1
  Constant_-1_74494/1 -> Product_2faf8/1
  State_Px_2_SG_D_1_42d3f/1 -> Product_2faf8/2
  State_Px_1_SG_D_1_862b1/1 -> Add_6853f/1
  Product_e53b9/1 -> Add_6853f/2
  Add_6853f/1 -> Divide_d781c/1
  Product_2faf8/1 -> Divide_6a425/1
  Constant_T_1_7fbbd/1 -> Divide_6a425/2
  Constant_T_1_c3252/1 -> Divide_d781c/2
  Divide_d781c/1 -> Add_d978a/2
  Add_d978a/1 -> Blockout_d_Px_2_SG_D_1_42534/1

== system IEEE9Buses/SG_D_1/d_Px_3_SG_D_1_block ==
  note: d_Px_3_SG_D_1 in SG9
      | $\frac{\mathrm{Px}_{2,\mathrm{SG},D,1}+T_{4}\,\left(\frac{\mathrm{Px}_{1,\mathrm{SG},D,1}-T_{2}\,\left(\frac{\mathrm{Px}_{1,\mathrm{SG},D,1}}{T_{w}}-\frac{w_{\mathrm{SG},D,1}-2\,\pi \,f_{0}}{T_{w}}\right)}{T_{1}}-\frac{\mathrm{Px}_{2,\mathrm{SG},D,1}}{T_{1}}\right)}{T_{3}}-\frac{\mathrm{Px}_{3,\mathrm{SG},D,1}}{T_{3}}$
      | Automatically generated on 2025-09-12 21:31:36 .
  State_Px_3_SG_D_1_8bd18 : Inport
  State_Px_2_SG_D_1_7ed7d : Inport  Port=2
  State_Px_2_SG_D_1_8a060 : Inport  Port=3
  State_Px_1_SG_D_1_12e65 : Inport  Port=4
  State_Px_1_SG_D_1_8beee : Inport  Port=5
  State_w_SG_D_1_841ae : Inport  Port=6
  Add_55b9b : Sum
  Add_7133e : Sum
  Add_8e9e9 : Sum
  Add_9656d : Sum
  Add_974d3 : Sum
  Add_ada35 : Sum
  Constant_-1_641e0 : Constant  Value=-1
  Constant_-1_cbc5f : Constant  Value=-1
  Constant_-1_f4b90 : Constant  Value=-1
  Constant_-2.0_4d915 : Constant  Value=-2.0
  Constant_T_1_06ee7 : Constant  Value=T_1
  Constant_T_1_711c0 : Constant  Value=T_1
  Constant_T_2_4e83b : Constant  Value=T_2
  Constant_T_3_40642 : Constant  Value=T_3
  Constant_T_3_acef4 : Constant  Value=T_3
  Constant_T_4_c758c : Constant  Value=T_4
  Constant_T_w_25e14 : Constant  Value=T_w
  Constant_T_w_3debf : Constant  Value=T_w
  Constant_f0_89783 : Constant  Value=f0
  Constant_pi_0690c : Constant  Value=pi
  Divide_16f2b : Product  Inputs=*/
  Divide_3521d : Product  Inputs=*/
  Divide_4621d : Product  Inputs=*/
  Divide_603e4 : Product  Inputs=*/
  Divide_9cb19 : Product  Inputs=*/
  Divide_bbe74 : Product  Inputs=*/
  Product_21b79 : Product
  Product_3843f : Product
  Product_5306d : Product
  Product_71171 : Product
  Product_735a7 : Product
  Product_8bb1c : Product
  Product_b6115 : Product
  Blockout_d_Px_3_SG_D_1_5e87f : Outport
  wires:
  Constant_T_w_25e14/1 -> Divide_16f2b/2
  Constant_-1_cbc5f/1 -> Product_21b79/1
  Add_7133e/1 -> Blockout_d_Px_3_SG_D_1_5e87f/1
  Constant_-2.0_4d915/1 -> Product_71171/1
  State_w_SG_D_1_841ae/1 -> Add_55b9b/2
  Constant_f0_89783/1 -> Product_b6115/2
  State_Px_1_SG_D_1_8beee/1 -> Product_21b79/2
  Constant_pi_0690c/1 -> Product_71171/2
  Product_b6115/1 -> Add_55b9b/1
  Product_71171/1 -> Product_b6115/1
  Product_21b79/1 -> Divide_16f2b/1
  Divide_4621d/1 -> Add_7133e/1
  Constant_T_3_acef4/1 -> Divide_9cb19/2
  Add_55b9b/1 -> Divide_bbe74/1
  Constant_T_w_3debf/1 -> Divide_bbe74/2
  Divide_16f2b/1 -> Add_8e9e9/1
  Divide_bbe74/1 -> Add_8e9e9/2
  Constant_-1_641e0/1 -> Product_5306d/1
  Constant_T_2_4e83b/1 -> Product_735a7/1
  Add_8e9e9/1 -> Product_735a7/2
  Constant_-1_f4b90/1 -> Product_8bb1c/1
  Divide_9cb19/1 -> Add_7133e/2
  Constant_T_3_40642/1 -> Divide_4621d/2
  State_Px_2_SG_D_1_8a060/1 -> Product_8bb1c/2
  State_Px_1_SG_D_1_12e65/1 -> Add_ada35/1
  Divide_603e4/1 -> Add_974d3/1
  Product_735a7/1 -> Add_ada35/2
  Product_8bb1c/1 -> Divide_603e4/1
  Product_5306d/1 -> Divide_4621d/1
  Constant_T_1_711c0/1 -> Divide_603e4/2
  Add_ada35/1 -> Divide_3521d/1
  Constant_T_1_06ee7/1 -> Divide_3521d/2
  Divide_3521d/1 -> Add_974d3/2
  Constant_T_4_c758c/1 -> Product_3843f/1
  Add_974d3/1 -> Product_3843f/2
  State_Px_3_SG_D_1_8bd18/1 -> Product_5306d/2
  State_Px_2_SG_D_1_7ed7d/1 -> Add_9656d/1
  Product_3843f/1 -> Add_9656d/2
  Add_9656d/1 -> Divide_9cb19/1

== system IEEE9Buses/SG_D_1/d_R_f_SG_D_1_block ==
  note: d_R_f_SG_D_1 in SG9
      | $-\frac{R_{f,\mathrm{SG},D,1}-\frac{E_{\mathrm{fd},\mathrm{SG},D,1}\,K_{F}}{T_{F}}}{T_{F}}$
      | Automatically generated on 2025-09-12 21:31:29 .
  State_E_fd_SG_D_1_36333 : Inport
  State_R_f_SG_D_1_cc465 : Inport  Port=2
  Constant_K_F_e1fd8 : Constant  Value=K_F
  Constant_T_F_06f29 : Constant  Value=T_F
  Constant_T_F_eb633 : Constant  Value=T_F
  Divide_4f78a : Product  Inputs=*/
  Divide_f3711 : Product  Inputs=*/
  Product_87820 : Product
  Subtract_e0979 : Sum  Inputs=+-
  Blockout_d_R_f_SG_D_1_13d30 : Outport
  wires:
  Constant_K_F_e1fd8/1 -> Product_87820/2
  Product_87820/1 -> Divide_f3711/1
  State_E_fd_SG_D_1_36333/1 -> Product_87820/1
  State_R_f_SG_D_1_cc465/1 -> Subtract_e0979/2
  Constant_T_F_eb633/1 -> Divide_f3711/2
  Divide_f3711/1 -> Subtract_e0979/1
  Divide_4f78a/1 -> Blockout_d_R_f_SG_D_1_13d30/1
  Subtract_e0979/1 -> Divide_4f78a/1
  Constant_T_F_06f29/1 -> Divide_4f78a/2

== system IEEE9Buses/SG_D_1/d_T_m_SG_D_1_block ==
  note: d_T_m_SG_D_1 in SG9
      | $-\frac{T_{m,\mathrm{SG},D,1}-T_{0}+\frac{\mathrm{SpeedPara}\,\left(w_{\mathrm{SG},D,1}-w_{\mathrm{ref}}\right)}{2\,f_{0}\,\pi }}{T_{\mathrm{speed}}}$
      | Automatically generated on 2025-09-12 21:31:20 .
  State_w_SG_D_1_aacae : Inport
  State_T_m_SG_D_1_00082 : Inport  Port=2
  Add_15a10 : Sum
  Add_3cc46 : Sum
  Constant_-1_6ef88 : Constant  Value=-1
  Constant_2.0_f873b : Constant  Value=2.0
  Constant_SpeedPara_64705 : Constant  Value=SpeedPara
  Constant_T_0_fa78d : Constant  Value=T_0
  Constant_T_speed_eb0f7 : Constant  Value=T_speed
  Constant_f0_2a0cd : Constant  Value=f0
  Constant_pi_4f214 : Constant  Value=pi
  Constant_w_ref_bdaf8 : Constant  Value=w_ref
  Divide_0bec3 : Product  Inputs=*/
  Divide_3af3e : Product  Inputs=*/
  Product_8a900 : Product
  Product_8dc05 : Product
  Product_ce9a8 : Product
  Product_fb348 : Product
  Subtract_53e1a : Sum  Inputs=+-
  Blockout_d_T_m_SG_D_1_f7f20 : Outport
  wires:
  Constant_-1_6ef88/1 -> Product_ce9a8/1
  Constant_w_ref_bdaf8/1 -> Add_15a10/2
  State_w_SG_D_1_aacae/1 -> Product_ce9a8/2
  Add_3cc46/1 -> Subtract_53e1a/1
  Add_15a10/1 -> Product_fb348/2
  Product_ce9a8/1 -> Add_15a10/1
  Constant_2.0_f873b/1 -> Product_8dc05/1
  Constant_pi_4f214/1 -> Product_8dc05/2
  Constant_SpeedPara_64705/1 -> Product_fb348/1
  Product_8dc05/1 -> Product_8a900/1
  Constant_f0_2a0cd/1 -> Product_8a900/2
  Constant_T_speed_eb0f7/1 -> Divide_0bec3/2
  Product_fb348/1 -> Divide_3af3e/1
  Product_8a900/1 -> Divide_3af3e/2
  Divide_3af3e/1 -> Add_3cc46/1
  Constant_T_0_fa78d/1 -> Add_3cc46/2
  State_T_m_SG_D_1_00082/1 -> Subtract_53e1a/2
  Subtract_53e1a/1 -> Divide_0bec3/1
  Divide_0bec3/1 -> Blockout_d_T_m_SG_D_1_f7f20/1
